simulink model "MOD5_tf"  (R2017a)
settings: Solver=FixedStepAuto  StartTime=0.0  StopTime=10  FixedStep=1/160000  RelTol=1e-3
undefined symbols (not defined in the file): H
libraries: dspmlti4 x2
settings Model: Creator=bhannigan  LastModifiedBy=bhannigan

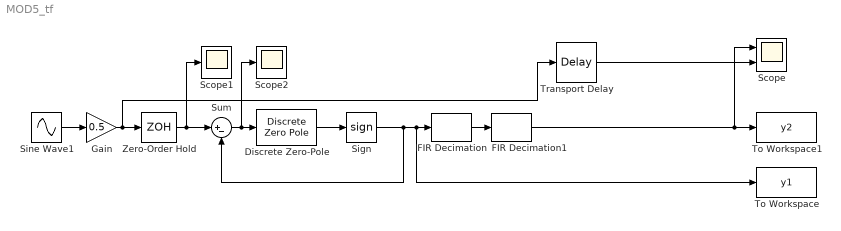
== system MOD5_tf ==
  Discrete Zero-Pole : DiscreteZeroPole  Zeros=H.Z{1}  Poles=H.P{1}  Gain=H.K  SampleTime=-1
  FIR Decimation : dspmlti4/FIR Decimation  FilterSource=Dialog parameters  h=fir1(31,1/64)  D=8  filtStruct=Direct form  FilterObject=FDECIM  framing=Allow multirate processing  inputOffset=0  outputBufInitCond=0  roundingMode=Floor  overflowMode=off  firstCoeffDataTypeStr=Inherit: Same word length as input  firstCoeffMin=[]  firstCoeffMax=[]  firstCoeffLastDataTypeStr=Inherit: Same word length as input  outputDataTypeStr=Inherit: Same as accumulator  outputMin=[]  outputMax=[]  outputLastDataTypeStr=Inherit: Same as accumulator
  FIR Decimation1 : dspmlti4/FIR Decimation  FilterSource=Dialog parameters  h=fir1(31,1/64)  D=8  filtStruct=Direct form  FilterObject=FDECIM  framing=Allow multirate processing  inputOffset=0  outputBufInitCond=0  roundingMode=Floor  overflowMode=off  firstCoeffDataTypeStr=Inherit: Same word length as input  firstCoeffMin=[]  firstCoeffMax=[]  firstCoeffLastDataTypeStr=Inherit: Same word length as input  outputDataTypeStr=Inherit: Same as accumulator  outputMin=[]  outputMax=[]  outputLastDataTypeStr=Inherit: Same as accumulator
  Gain : Gain  Gain=0.5
  Scope : Scope  NumInputPorts=2
  Scope1 : Scope
  Scope2 : Scope
  Sign : Signum
  Sine Wave1 : Sin  Frequency=2*pi*100  SampleTime=0
  Sum : Sum  Inputs=|+-
  To Workspace : ToWorkspace  VariableName=y1  SaveFormat=Timeseries  SampleTime=-1
  To Workspace1 : ToWorkspace  VariableName=y2  SaveFormat=Timeseries  SampleTime=-1
  Transport Delay : TransportDelay  DelayTime=126/160000
  Zero-Order Hold : ZeroOrderHold  SampleTime=1/160000
  wires:
  Sum/1 -> Scope2/1, Discrete Zero-Pole/1
  Discrete Zero-Pole/1 -> Sign/1
  Gain/1 -> Transport Delay/1, Zero-Order Hold/1
  Zero-Order Hold/1 -> Sum/1, Scope1/1
  Sign/1 -> Sum/2, To Workspace/1, FIR Decimation/1
  Sine Wave1/1 -> Gain/1
  FIR Decimation/1 -> FIR Decimation1/1
  FIR Decimation1/1 -> To Workspace1/1, Scope/1
  Transport Delay/1 -> Scope/2
